simulink model "BDC_motor"  (R2015b)
settings: Solver=VariableStepAuto  StartTime=0.0  StopTime=10.0  RelTol=1e-3
settings Model: Creator=Meghdeep  LastModifiedBy=Meghdeep

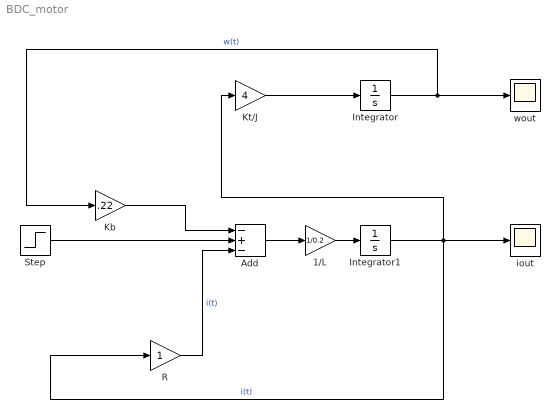
== system BDC_motor ==
  "1/L " : Gain  Gain=1/0.2
  Add : Sum  Inputs=-+-
  Integrator : Integrator
  Integrator1 : Integrator
  "Kb " : Gain  Gain=.22
  "Kt/J " : Gain  Gain=4
  R : Gain
  Step : Step  SampleTime=0
  "iout " : Scope
  wout : Scope
  wires:
  Integrator/1 -> wout/1, "Kb "/1  "w(t)"
  Integrator1/1 -> "iout "/1, R/1, "Kt/J "/1  "i(t)"
  "Kt/J "/1 -> Integrator/1
  Step/1 -> Add/2
  R/1 -> Add/3  "i(t)"
  Add/1 -> "1/L "/1
  "Kb "/1 -> Add/1
  "1/L "/1 -> Integrator1/1
